simulink model "SecRwLtStFwdBkwdCtrl"  (R2024b)
settings: Solver=FixedStepDiscrete  StartTime=0.0  StopTime=10.0  FixedStep=0.01  RelTol=1e-3
undefined symbols (not defined in the file or in its folder): KeSMSuMdMotFinshdTm_Val, KeSMSuMdRetryTm1_Val, KeSMSuModeReqDurgTm_Val
libraries: StCtrlLibBkRecln x1
settings Model: Creator=sn2xws  LastModifiedBy=sn55gm
settings Model: ModifiedHistory=|
  | 2024.10.14 V3.0.0 bitmask接口改为变量接口
  | 25.7.7 V3.13.0 Md61 Md62新增Retry口
  | 25.12.04 V3.14.0 md10防夹后退出
settings SolverCC: AlgebraicLoopSolver=TrustRegion
settings DataIOCC: SaveFormat=StructureWithTime  ReturnWorkspaceOutputs=off
settings OptimizationCC: DefaultParameterBehavior=Inlined  EnhancedBackFolding=on  PassReuseOutputArgsAs=Individual arguments  ZeroExternalMemoryAtStartup=off  ZeroInternalMemoryAtStartup=off  OptimizeBlockOrder=speed  DifferentSizesBufferReuse=on  OptimizationCustomize=off  EfficientTunableParamExpr=on
settings DebuggingCC: ParameterTunabilityLossMsg=error  UnconnectedInputMsg=warning  UnconnectedOutputMsg=warning  UnconnectedLineMsg=warning  ArithmeticOperatorsInVariantConditions=warning
settings ModelReferenceCC: EnableRefExpFcnMdlSchedulingChecks=on  ModelReferenceNumInstancesAllowed=Single
settings SFSimCC: MATLABDynamicMemAlloc=off  CustomCodeUndefinedFunction=UseInterfaceOnly
settings RTWCC: Description=AUTOSAR  SystemTargetFile=autosar.tlc  GenCodeOnly=on  TemplateMakefile=ert_default_tmf  GenerateReport=on  IncludeHyperlinkInReport=on  LaunchReport=on  DataTypeReplacement=CDataTypesFixedWidth  GenerateTraceInfo=on  GenerateTraceReport=on  GenerateTraceReportSl=on  GenerateTraceReportSf=on  GenerateTraceReportEml=on  GenerateCodeMetricsReport=on  GPUComputeCapability=3.5
settings CodeAppCC: ForceParamTrailComments=on  IgnoreCustomStorageClasses=off  OperatorAnnotations=on  SimulinkDataObjDesc=on  SFDataObjDesc=on  InsertBlockDesc=on
settings STFCustomTargetCC: TargetLangStandard=C99 (ISO)  MultiwordLength=256  ParMdlRefBuildCompliant=on  CompOptLevelCompliant=on  IncludeMdlTerminateFcn=off  CombineOutputUpdateFcns=on  SuppressErrorStatus=on  ERTCustomFileBanners=on  SupportNonFinite=off  SupportComplex=off  SupportContinuousTime=off  SupportNonInlinedSFcns=off  RemoveResetFunc=on  MATLABClassNameForMDSCustomization=Simulink.SoftwareTarget.ERTCustomization  AutosarCompliant=on  UseToolchainInfoCompliant=on  LookupTableObjectStructAxisOrder=2,1,3,4,...  LUTObjectStructOrderEvenSpacing=Size,Table,Breakpoints  SystemTargetFile=autosar.tlc
settings ERTTargetCC: TargetLangStandard=C99 (ISO)  ConcurrentExecutionCompliant=off  IncludeMdlTerminateFcn=off  SuppressErrorStatus=on  SupportNonFinite=off  SupportComplex=off  ModelStepFunctionPrototypeControlCompliant=off  CPPClassGenCompliant=off  AutosarCompliant=on  LookupTableObjectStructAxisOrder=2,1,3,4,...  LUTObjectStructOrderEvenSpacing=Size,Table,Breakpoints  ERTCustomFileTemplate=example_file_process.tlc  ERTFilePackagingFormat=Compact  BooleanTrueId=TRUE  BooleanFalseId=FALSE  DynamicArrayContainerType=coder::array

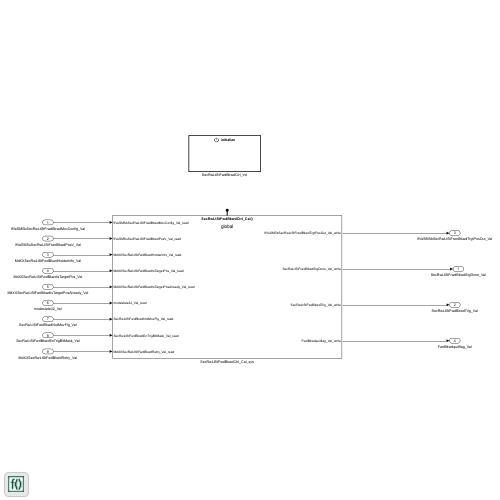
[thumbnail: Simulink's stored preview of the top-level diagram]
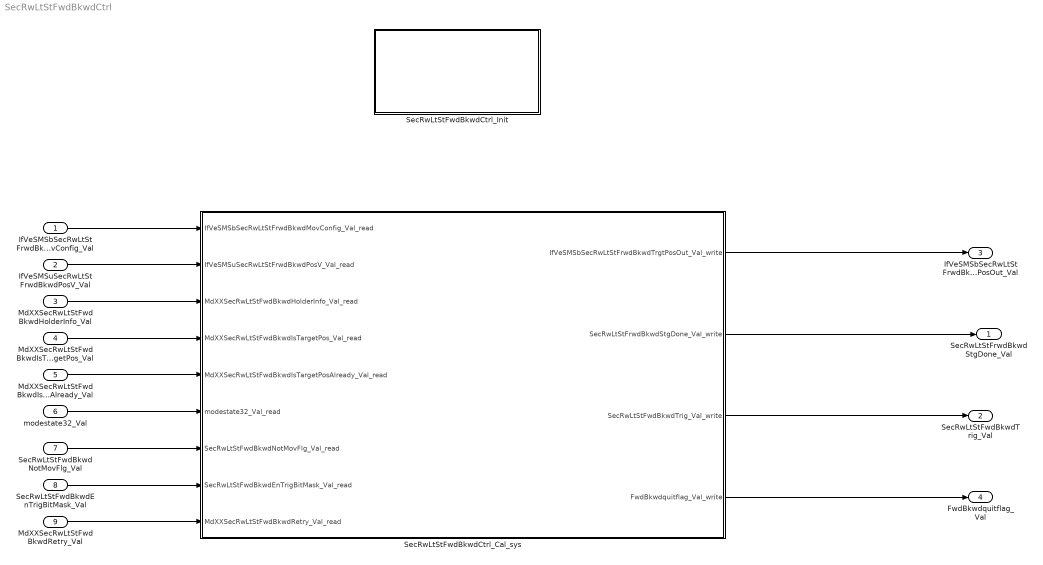
== system SecRwLtStFwdBkwdCtrl ==
  IfVeSMSbSecRwLtStFrwdBkwdMovConfig_Val : Inport  OutDataTypeStr=boolean  PortDimensions=1
  IfVeSMSuSecRwLtStFrwdBkwdPosV_Val : Inport  Port=2  OutDataTypeStr=boolean  PortDimensions=1
  MdXXSecRwLtStFwdBkwdHolderInfo_Val : Inport  Port=3  OutDataTypeStr=uint32  PortDimensions=1
  MdXXSecRwLtStFwdBkwdIsTargetPos_Val : Inport  Port=4  OutDataTypeStr=uint32  PortDimensions=1
  MdXXSecRwLtStFwdBkwdIsTargetPosAlready_Val : Inport  Port=5  OutDataTypeStr=uint32  PortDimensions=1
  modestate32_Val : Inport  Port=6  OutDataTypeStr=uint32  PortDimensions=1
  SecRwLtStFwdBkwdNotMovFlg_Val : Inport  Port=7  OutDataTypeStr=boolean  PortDimensions=1
  SecRwLtStFwdBkwdEnTrigBitMask_Val : Inport  Port=8  OutDataTypeStr=uint32  PortDimensions=1
  MdXXSecRwLtStFwdBkwdRetry_Val : Inport  Port=9  OutDataTypeStr=uint32  PortDimensions=1
  SecRwLtStFwdBkwdCtrl_Cal_sys : Subsystem
  SecRwLtStFwdBkwdCtrl_Init : Subsystem
  SecRwLtStFrwdBkwdStgDone_Val : Outport  OutDataTypeStr=boolean  PortDimensions=1  VectorParamsAs1DForOutWhenUnconnected=off
  SecRwLtStFwdBkwdTrig_Val : Outport  Port=2  OutDataTypeStr=boolean  PortDimensions=1  VectorParamsAs1DForOutWhenUnconnected=off
  IfVeSMSbSecRwLtStFrwdBkwdTrgtPosOut_Val : Outport  Port=3  OutDataTypeStr=boolean  PortDimensions=1  VectorParamsAs1DForOutWhenUnconnected=off
  FwdBkwdquitflag_Val : Outport  Port=4  OutDataTypeStr=boolean  PortDimensions=1  VectorParamsAs1DForOutWhenUnconnected=off
  wires:
  IfVeSMSbSecRwLtStFrwdBkwdMovConfig_Val/1 -> SecRwLtStFwdBkwdCtrl_Cal_sys/1(IfVeSMSbSecRwLtStFrwdBkwdMovConfig_Val_read)
  IfVeSMSuSecRwLtStFrwdBkwdPosV_Val/1 -> SecRwLtStFwdBkwdCtrl_Cal_sys/2(IfVeSMSuSecRwLtStFrwdBkwdPosV_Val_read)
  MdXXSecRwLtStFwdBkwdHolderInfo_Val/1 -> SecRwLtStFwdBkwdCtrl_Cal_sys/3(MdXXSecRwLtStFwdBkwdHolderInfo_Val_read)
  MdXXSecRwLtStFwdBkwdIsTargetPos_Val/1 -> SecRwLtStFwdBkwdCtrl_Cal_sys/4(MdXXSecRwLtStFwdBkwdIsTargetPos_Val_read)
  MdXXSecRwLtStFwdBkwdIsTargetPosAlready_Val/1 -> SecRwLtStFwdBkwdCtrl_Cal_sys/5(MdXXSecRwLtStFwdBkwdIsTargetPosAlready_Val_read)
  modestate32_Val/1 -> SecRwLtStFwdBkwdCtrl_Cal_sys/6(modestate32_Val_read)
  SecRwLtStFwdBkwdNotMovFlg_Val/1 -> SecRwLtStFwdBkwdCtrl_Cal_sys/7(SecRwLtStFwdBkwdNotMovFlg_Val_read)
  SecRwLtStFwdBkwdCtrl_Cal_sys/1(IfVeSMSbSecRwLtStFrwdBkwdTrgtPosOut_Val_write) -> IfVeSMSbSecRwLtStFrwdBkwdTrgtPosOut_Val/1
  SecRwLtStFwdBkwdCtrl_Cal_sys/2(SecRwLtStFrwdBkwdStgDone_Val_write) -> SecRwLtStFrwdBkwdStgDone_Val/1
  SecRwLtStFwdBkwdCtrl_Cal_sys/3(SecRwLtStFwdBkwdTrig_Val_write) -> SecRwLtStFwdBkwdTrig_Val/1
  SecRwLtStFwdBkwdEnTrigBitMask_Val/1 -> SecRwLtStFwdBkwdCtrl_Cal_sys/8(SecRwLtStFwdBkwdEnTrigBitMask_Val_read)
  MdXXSecRwLtStFwdBkwdRetry_Val/1 -> SecRwLtStFwdBkwdCtrl_Cal_sys/9(MdXXSecRwLtStFwdBkwdRetry_Val_read)
  SecRwLtStFwdBkwdCtrl_Cal_sys/4(FwdBkwdquitflag_Val_write) -> FwdBkwdquitflag_Val/1

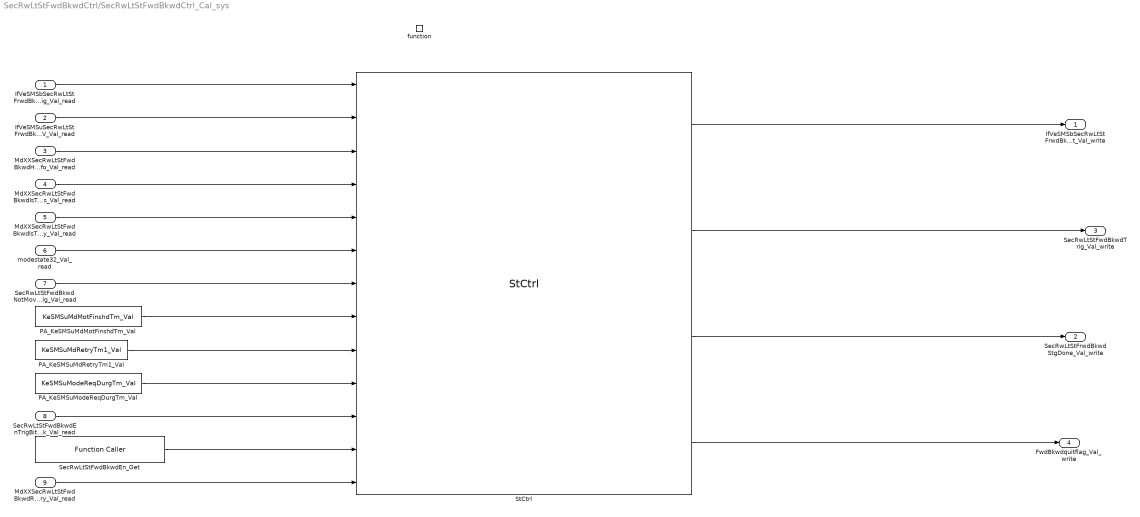
== system SecRwLtStFwdBkwdCtrl/SecRwLtStFwdBkwdCtrl_Cal_sys ==
  IfVeSMSbSecRwLtStFrwdBkwdMovConfig_Val_read : Inport
  IfVeSMSuSecRwLtStFrwdBkwdPosV_Val_read : Inport  Port=2
  MdXXSecRwLtStFwdBkwdHolderInfo_Val_read : Inport  Port=3
  MdXXSecRwLtStFwdBkwdIsTargetPos_Val_read : Inport  Port=4
  MdXXSecRwLtStFwdBkwdIsTargetPosAlready_Val_read : Inport  Port=5
  modestate32_Val_read : Inport  Port=6
  SecRwLtStFwdBkwdNotMovFlg_Val_read : Inport  Port=7
  SecRwLtStFwdBkwdEnTrigBitMask_Val_read : Inport  Port=8
  MdXXSecRwLtStFwdBkwdRetry_Val_read : Inport  Port=9
  function : TriggerPort  TriggerType=function-call  IsSimulinkFunction=on  FunctionName=SecRwLtStFwdBkwdCtrl_Cal  VariantControl=(inherit)
  PA_KeSMSuMdMotFinshdTm_Val : Constant  Value=KeSMSuMdMotFinshdTm_Val
  PA_KeSMSuMdRetryTm1_Val : Constant  Value=KeSMSuMdRetryTm1_Val
  PA_KeSMSuModeReqDurgTm_Val : Constant  Value=KeSMSuModeReqDurgTm_Val
  SecRwLtStFwdBkwdEn_Get : FunctionCaller  FunctionPrototype=data = SecRwLtStFwdBkwdEn_Get()  InputArgumentSpecifications=<Enter example>  OutputArgumentSpecifications=uint32(1)
  StCtrl : StCtrlLibBkRecln/StCtrl  SystemSampleTime=-1  VariantActivationTime=update diagram  AllowFlexibleInterface=on  Latency=0  AutoFrameSizeCalculation=off
  IfVeSMSbSecRwLtStFrwdBkwdTrgtPosOut_Val_write : Outport  VectorParamsAs1DForOutWhenUnconnected=off
      settings: EnsureOutportIsVirtual=on
  SecRwLtStFrwdBkwdStgDone_Val_write : Outport  Port=2  VectorParamsAs1DForOutWhenUnconnected=off
      settings: EnsureOutportIsVirtual=on
  SecRwLtStFwdBkwdTrig_Val_write : Outport  Port=3  VectorParamsAs1DForOutWhenUnconnected=off
      settings: EnsureOutportIsVirtual=on
  FwdBkwdquitflag_Val_write : Outport  Port=4  VectorParamsAs1DForOutWhenUnconnected=off
      settings: EnsureOutportIsVirtual=on
  wires:
  StCtrl/1 -> IfVeSMSbSecRwLtStFrwdBkwdTrgtPosOut_Val_write/1
  SecRwLtStFwdBkwdEnTrigBitMask_Val_read/1 -> StCtrl/11
  PA_KeSMSuMdMotFinshdTm_Val/1 -> StCtrl/8
  SecRwLtStFwdBkwdEn_Get/1 -> StCtrl/12
  PA_KeSMSuModeReqDurgTm_Val/1 -> StCtrl/10
  PA_KeSMSuMdRetryTm1_Val/1 -> StCtrl/9
  IfVeSMSbSecRwLtStFrwdBkwdMovConfig_Val_read/1 -> StCtrl/1
  IfVeSMSuSecRwLtStFrwdBkwdPosV_Val_read/1 -> StCtrl/2
  MdXXSecRwLtStFwdBkwdHolderInfo_Val_read/1 -> StCtrl/3
  MdXXSecRwLtStFwdBkwdIsTargetPos_Val_read/1 -> StCtrl/4
  MdXXSecRwLtStFwdBkwdIsTargetPosAlready_Val_read/1 -> StCtrl/5
  modestate32_Val_read/1 -> StCtrl/6
  SecRwLtStFwdBkwdNotMovFlg_Val_read/1 -> StCtrl/7
  StCtrl/2 -> SecRwLtStFwdBkwdTrig_Val_write/1
  StCtrl/3 -> SecRwLtStFrwdBkwdStgDone_Val_write/1
  MdXXSecRwLtStFwdBkwdRetry_Val_read/1 -> StCtrl/13
  StCtrl/4 -> FwdBkwdquitflag_Val_write/1

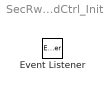
== system SecRwLtStFwdBkwdCtrl/SecRwLtStFwdBkwdCtrl_Init ==
  Event Listener : EventListener  EventName=reset
